simulink library "lib2"  (Simulink 6.0)
libraries: lib1 x1
settings Model: Creator=awarlock  LastModifiedBy=mshakeri  ExtModeAutoUpdateStatusClock=off

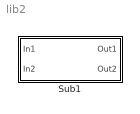
== system lib2 ==
  Sub1 : Subsystem  TreatAsAtomicUnit=on

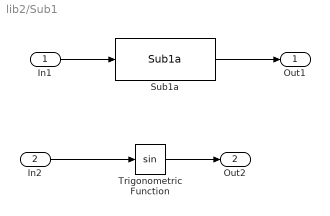
== system lib2/Sub1 ==
  In1 : Inport
  In2 : Inport  Port=2
  Sub1a : lib1/Sub1a  TreatAsAtomicUnit=on  SimViewingDevice=off  DataTypeOverride=UseLocalSettings  MinMaxOverflowLogging=UseLocalSettings
      settings: Permissions=ReadWrite  RTWFcnNameOpts=Auto  RTWFileNameOpts=Auto
  Trigonometric Function : Trigonometry
  Out1 : Outport
  Out2 : Outport  Port=2
  wires:
  In1/1 -> Sub1a/1
  Sub1a/1 -> Out1/1
  In2/1 -> Trigonometric Function/1
  Trigonometric Function/1 -> Out2/1
